simulink model "BHclientTORQUE"  (Simulink 7.4)
settings: Solver=ode3  StartTime=0.0  StopTime=inf  FixedStep=0.01  RelTol=1e-3
libraries: planmant x1
settings Model: Creator=Admin  LastModifiedBy=Admin

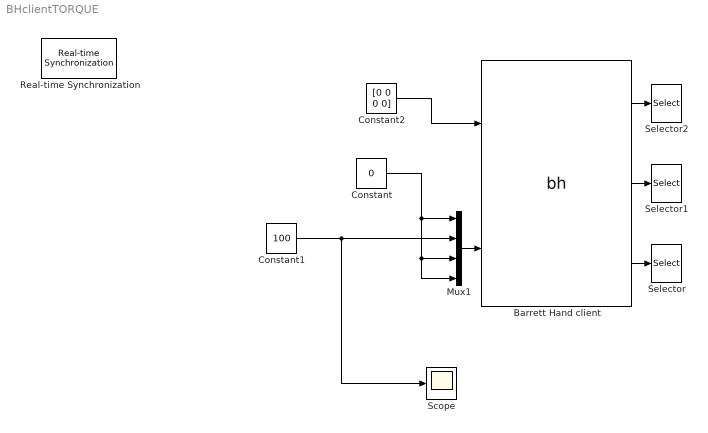
== system BHclientTORQUE ==
  Barrett Hand client : S-Function  FunctionName=bh  Parameters=IP port mode262 mode280 ST a0 a1 a2 a3 a4 a41 a5 a6 a7 a8 a81 a9  EnableBusSupport=off  mask(Barrett Hand UDP client){mode262=Velocity, mode280=Torque, IP=193.2.6.168, port=4444, ST=0.01, a0=off, a1=off, a2=off, a3=off, a4=off, a41=off, a5=on, a6=on, a7=off, a8=off, a81=on, a9=off}
      mask prompts: mode262 "BH262 mode"; mode280 "BH280 mode"; port "UDP port"; a0 "Time"; a1 "262 position"; a2 "262 velocity"; a3 "262 deltap"; a4 "262 strain"; a41 "262 strain filt"; a5 "280 position"; a6 "280 velocity"; a7 "280 deltap"; a8 "280 strain"; a81 "280 strain filt"; a9 "pps"
      mask help:
      | Make sure you select the right mode. Sending positions when velocity mode
      | selected may not end well.
      |
      | Units are rad and rad/s. Strain and pps data is raw (no units)
      mask StyleString: popup(Velocity|Position|Torque|Other),popup(Velocity|Position|Torque|Other),edit,edit,edit,checkbox,checkbox,checkbox,checkbox,checkbox,checkbox,checkbox,checkbox,checkbox,checkbox,checkbox,checkbox
      mask CallbackString: togglePorts()|togglePorts()|togglePorts()|togglePorts()||togglePorts()|togglePorts()|togglePorts()|togglePorts()|togglePorts()|togglePorts()|togglePorts()|togglePorts()|togglePorts()|togglePorts()|togglePorts()|togglePorts()
      mask TabNameString: Control,Control,Control,Control,Control,Outputs,Outputs,Outputs,Outputs,Outputs,Outputs,Outputs,Outputs,Outputs,Outputs,Outputs,Outputs
      mask Display: text(0.3, 0.9, '\fontsize{10}IP: {\bf193.2.6.168 \newline\rmport: \bf4444}', 'horizontalAlignment', 'center','texmode','on')color('red')port_label('input',1,'\fontsize{12}BH262 {\newline\bfVelocity}','texmode','on')color('green') port_label('input',2,'\fontsize{12}BH280 {\newline\bfTorque}','texmode','on')color('black')port_label('output',1,'\fontsize{11}BH280 {\bfPosition}','texmode','on');port_label('output',2,'BH280 {Velocity}','texmode','on');port_label('output',3,'BH280 {StrainFltr}','texmode','on');
  Constant : Constant  Value=0  OutDataType=fixdt(1, 16)  OutScaling=2^0
  Constant1 : Constant  Value=100  OutDataType=fixdt(1, 16)  OutScaling=2^0
  Constant2 : Constant  Value=[0 0 0 0]  OutDataType=fixdt(1, 16)  OutScaling=2^0
  Mux1 : Mux
  Real-time Synchronization : planmant/Utility/Real-time Synchronization  SystemSampleTime=-1
  Scope : Scope
  Selector : Selector  InputPortWidth=4  IndexOptions=Index vector (dialog)  Indices=2  OutputSizes=1
  Selector1 : Selector  InputPortWidth=4  IndexOptions=Index vector (dialog)  Indices=2  OutputSizes=1
  Selector2 : Selector  InputPortWidth=4  IndexOptions=Index vector (dialog)  Indices=2  OutputSizes=1
  wires:
  Mux1/1 -> Barrett Hand client/2
  Barrett Hand client/2 -> Selector1/1
  Barrett Hand client/1 -> Selector2/1
  Barrett Hand client/3 -> Selector/1
  Constant/1 -> Mux1/3, Mux1/4, Mux1/1
  Constant1/1 -> Mux1/2, Scope/1
  Constant2/1 -> Barrett Hand client/1
